simulink model "anc1_lms"  (R2013a)
settings: Solver=VariableStepDiscrete  StartTime=0.0  StopTime=10  RelTol=1e-3
libraries: simulink x1
settings Model: Creator=balazs.varga  LastModifiedBy=balazs.varga

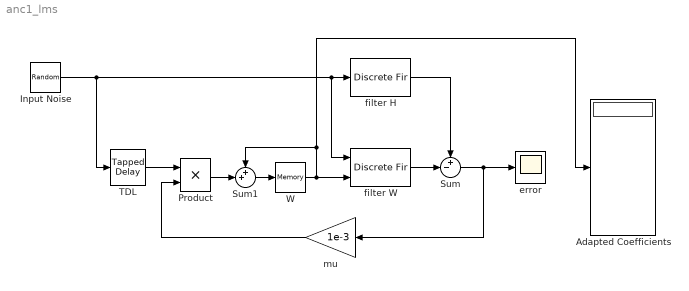
== system anc1_lms ==
  Adapted Coefficients : Display
  Input Noise : RandomNumber  Variance=0.1  SampleTime=1e-4
  Product : Product  SampleTime=1e-4
  Sum : Sum  Inputs=+-|  SampleTime=1e-4
  Sum1 : Sum  Inputs=++|  SampleTime=1e-4
  TDL : simulink/Discrete/Tapped Delay  vinit=0.0  samptime=1e-4  NumDelays=9  DelayOrder=Newest  includeCurrent=on
  W : Memory  X0=zeros(1,10)  InheritSampleTime=on
  error : Scope
      settings: YMin=-0.45  YMax=0.45
  filter H : DiscreteFir  Coefficients=[1 2 3 4 5]  SampleTime=1e-4
  filter W : DiscreteFir  CoefSource=Input port  SampleTime=1e-4
  "mu " : Gain  Gain=1e-3  SampleTime=1e-4
  wires:
  W/1 -> filter W/2, Adapted Coefficients/1, Sum1/1
  filter W/1 -> Sum/2
  filter H/1 -> Sum/1
  TDL/1 -> Product/1
  Sum/1 -> "mu "/1, error/1
  Sum1/1 -> W/1
  Product/1 -> Sum1/2
  Input Noise/1 -> TDL/1, filter W/1, filter H/1
  "mu "/1 -> Product/2
